simulink model "buck"  (R2024b)
settings: Solver=VariableStepAuto  StartTime=0.0  StopTime=delay*2000  RelTol=1e-3
InitFcn:
  | run('../matlab_code/parameters.m')
undefined symbols (not defined in the file or in its folder): buck_freq, Cin, Lout
libraries: spsCurrentMeasurementLib x4, spsSeriesRLCBranchLib x3, spsDiodeLib x2, spsMosfetLib x2, spsVoltageMeasurementLib x2, spsDCVoltageSourceLib x1, spsPVArrayLib x1, sps_lib x1
settings Model: LastModifiedBy=deso

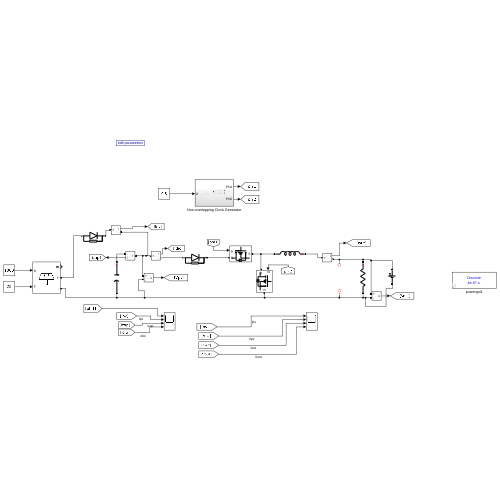
[thumbnail: Simulink's stored preview of the top-level diagram]
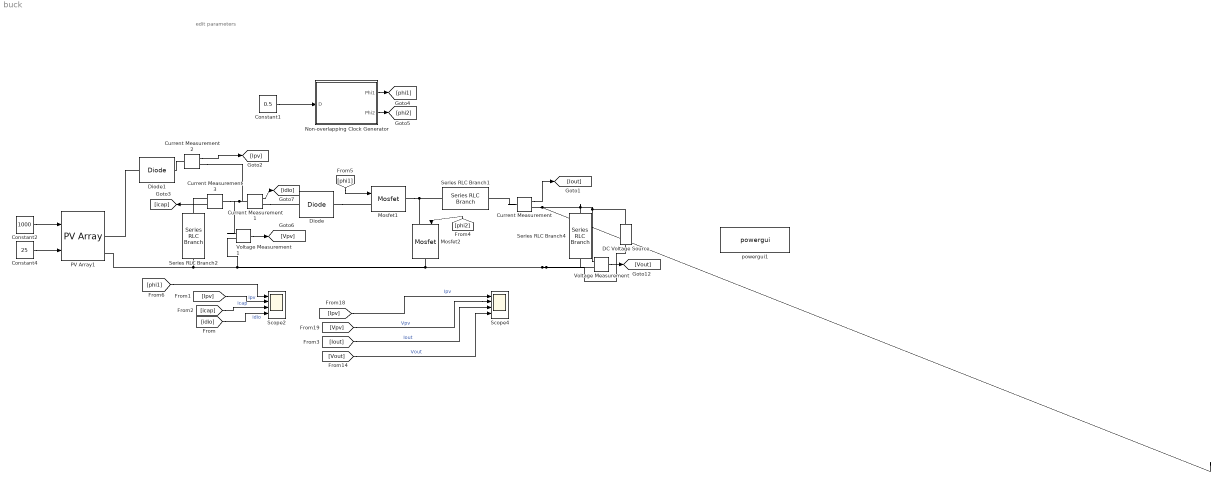
== system buck ==
  note: edit parameters
  Constant1 : Constant  Value=0.5
  Constant2 : Constant  Value=1000
  Constant4 : Constant  Value=25
  Current Measurement{,1..3} (4 alike) : spsCurrentMeasurementLib/Current Measurement  PhasorSimulation=off  OutputType=Complex  PSBequivalent=0
  DC Voltage Source : spsDCVoltageSourceLib/DC Voltage Source  Amplitude=5  Measurements=None
  Diode : spsDiodeLib/Diode  Ron=0.001  Lon=0  Vf=0.5  IC=0  UseSnubber=0  Rs=500  Cs=250e-9  Measurements=off
  Diode1 : spsDiodeLib/Diode  Ron=0.001  Lon=0  Vf=0.5  IC=0  UseSnubber=0  Rs=500  Cs=250e-9  Measurements=off
  Mosfet1 : spsMosfetLib/Mosfet  Ron=10e-3  Lon=1e-9  Rd=0.01  Vfd=0.7  IC=0  Rs=1e5  Cs=inf  Measurements=off
  Mosfet2 : spsMosfetLib/Mosfet  Ron=10e-3  Lon=1e-9  Rd=0.01  Vfd=0.7  IC=0  Rs=1e5  Cs=inf  Measurements=off
  Non-overlapping Clock Generator : Subsystem
  PV Array1 : spsPVArrayLib/PV Array  Npar=1  Nser=1  PlotType=one module @ 25 deg.C & specified irradiances  S_vec="[ 1000  500  100 ]"  Temp_C_vec="[ 45 25  ]"  ModuleName=A10Green Technology A10J-M60-235  PlotWhenSelected=off  Pm=235.008  Ncell=60  Voc=36.72  Isc=8.23  Vm=30.6  Im=7.68  beta_Voc_pc=-0.359  alpha_Isc_pc=0.096999  beta_Voc=-0.13182  alpha_Isc=0.007983  IL=8.2383  I0=2.8335e-10  nI=0.98962  Rsh=196.9278  Rs=0.19811  RobustModel=off  RobustCellTemperature=313.3991  BAL=on  Tc=1e-6  Tfilter=5e-5
  Scope2 : Scope  NumInputPorts=4
  Scope4 : Scope  NumInputPorts=4
  Series RLC Branch1 : spsSeriesRLCBranchLib/Series RLC Branch  LConnTagsString=__new0  RConnTagsString=__new0  BranchType=L  Resistance=0  Inductance=Lout  SetiL0=off  InitialCurrent=0  Capacitance=100e-6  Setx0=off  InitialVoltage=0  Measurements=None
  Series RLC Branch2 : spsSeriesRLCBranchLib/Series RLC Branch  LConnTagsString=__new0  RConnTagsString=__new0  BranchType=C  Resistance=0  Inductance=1e-6  SetiL0=off  InitialCurrent=0  Capacitance=Cin  Setx0=off  InitialVoltage=0  Measurements=None
  Series RLC Branch4 : spsSeriesRLCBranchLib/Series RLC Branch  LConnTagsString=__new0  RConnTagsString=__new0  BranchType=R  Resistance=1e0  Inductance=1e-6  SetiL0=off  InitialCurrent=0  Capacitance=Cin  Setx0=off  InitialVoltage=0  Measurements=None
  Voltage Measurement : spsVoltageMeasurementLib/Voltage Measurement  PhasorSimulation=off  OutputType=Complex  PSBequivalent=0
  Voltage Measurement1 : spsVoltageMeasurementLib/Voltage Measurement  PhasorSimulation=off  OutputType=Complex  PSBequivalent=0
  powergui1 : sps_lib/powergui  Priority=1  SimulationMode=Discrete  SampleTime=1/(25*buck_freq)  frequency=60  Iterations=50  frequencyindice=0  Pbase=100e6  ErrMax=1e-4  UnitsV=kV  UnitsW=MW  buscounter=0  FunctionMessages=off  echomessages=off  EnableUseOfTLC=off  CurrentSourceSwitches=off  DisableSnubberDevices=off  DisableRonSwitches=off  DisableVfSwitches=off  DisplayEquations=off  AutomaticDiscreteSolvers=off  SolverType=Tustin/Backward Euler (TBE)  Interpol=off  ExternalGateDelay=off  methode=off  Ts=100  x0status=blocks  SPID=on  SwTol=0  HookPort=off  NonlinearTolerance=1e-4  nMaxIteration=100  ContinueOnMaxIteration=off  RestoreLinks=warning  ResistiveCurrentMeasurement=off  Frange=[0:2:500]  Ylog=off  Xlog=on  ShowGrid=off  save=off  variable=ZData  structure=0  ZoomFFT=off  StartTime=0.0  cycles=1  DisplayStyle=1  fundamental=60  FreqAxis=off  MaxFrequency=1000  frequencyindicesteady=1  RmsSteady=1  display=off
  wires:
  Non-overlapping Clock Generator/2(Phi2) -> [phi2]
  Non-overlapping Clock Generator/1(Phi1) -> [phi1]
  Constant4/1 -> PV Array1/2
  [phi2] -> Mosfet2/1
  [phi1] -> Mosfet1/1
  Constant2/1 -> PV Array1/1
  [Ipv] -> Scope4/1  "Ipv"
  [Vpv] -> Scope4/2  "Vpv"
  [Iout] -> Scope4/3  "Iout"
  [Vout] -> Scope4/4  "Vout"
  Voltage Measurement/1 -> [Vout]
  Current Measurement/1 -> [Iout]
  Voltage Measurement1/1 -> [Vpv]
  Current Measurement1/1 -> [idio]
  Constant1/1 -> Non-overlapping Clock Generator/1(D)
  Current Measurement2/1 -> [Ipv]
  Current Measurement3/1 -> [icap]
  [idio] -> Scope2/4  "idio"
  [icap] -> Scope2/3  "icap"
  [Ipv] -> Scope2/2  "Ipv"
  [phi1] -> Scope2/1
  connections:
  Series RLC Branch4/RConn1 -- DC Voltage Source/LConn1 -- Voltage Measurement/LConn2 -- Mosfet2/RConn1 -- Series RLC Branch2/RConn1 -- PV Array1/RConn2 -- Voltage Measurement1/LConn2
  Diode/RConn1 -- Mosfet1/LConn1
  Diode1/LConn1 -- PV Array1/RConn1
  Mosfet1/RConn1 -- Series RLC Branch1/RConn1 -- Mosfet2/LConn1
  Current Measurement/LConn1 -- Series RLC Branch1/LConn1
  Current Measurement/RConn1 -- Series RLC Branch4/LConn1 -- DC Voltage Source/RConn1 -- Voltage Measurement/LConn1
  Current Measurement1/RConn1 -- Diode/LConn1
  Current Measurement1/LConn1 -- Voltage Measurement1/LConn1 -- Current Measurement3/LConn1 -- Current Measurement2/RConn1
  Current Measurement2/LConn1 -- Diode1/RConn1
  Current Measurement3/RConn1 -- Series RLC Branch2/LConn1

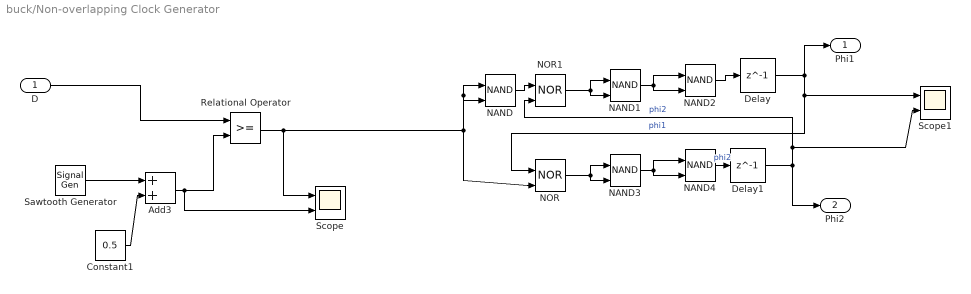
== system buck/Non-overlapping Clock Generator ==
  D : Inport
  Add3 : Sum
  Constant1 : Constant  Value=0.5
  Delay : Delay  DelayLength=1  SampleTime=1/(buck_freq*100)
  Delay1 : Delay  DelayLength=1  SampleTime=1/(buck_freq*100)
  NAND{,1..4} (5 alike) : Logic  Operator=NAND  IconShape=distinctive  AllPortsSameDT=off  OutDataTypeStr=boolean
  NOR : Logic  Operator=NOR  IconShape=distinctive  AllPortsSameDT=off  OutDataTypeStr=boolean
  NOR1 : Logic  Operator=NOR  IconShape=distinctive  AllPortsSameDT=off  OutDataTypeStr=boolean
  Relational Operator : RelationalOperator  OutDataTypeStr=boolean  RndMeth=Simplest  InputSameDT=off
  Sawtooth Generator : SignalGenerator  WaveForm=sawtooth  Amplitude=-0.5  Frequency=buck_freq
  Scope : Scope  NumInputPorts=2
  Scope1 : Scope  NumInputPorts=2
  Phi1 : Outport
  Phi2 : Outport  Port=2
  wires:
  NOR/1 -> NAND3/1, NAND3/2
  NAND3/1 -> NAND4/1, NAND4/2
  NAND/1 -> NOR1/1
  NOR1/1 -> NAND1/1, NAND1/2
  Delay1/1 -> NOR1/2, Scope1/2, Phi2/1  "phi2"
  NAND2/1 -> Delay/1
  Delay/1 -> NOR/1, Scope1/1, Phi1/1  "phi1"
  NAND1/1 -> NAND2/1, NAND2/2
  Relational Operator/1 -> NOR/2, NAND/2, NAND/1, Scope/1
  Constant1/1 -> Add3/2
  Sawtooth Generator/1 -> Add3/1
  Add3/1 -> Scope/2, Relational Operator/2
  D/1 -> Relational Operator/1
  NAND4/1 -> Delay1/1  "phi2"
